simulink model "Example4"  (R2020a)
settings: Solver=ode15s  StartTime=0.0  StopTime=0.2  FixedStep=0.01  RelTol=1e-3
undefined symbols (not defined in the file): b, J, K, L, R
settings Model: DataDictionary=motor_data.sldd  Creator=aishw  LastModifiedBy=aishw

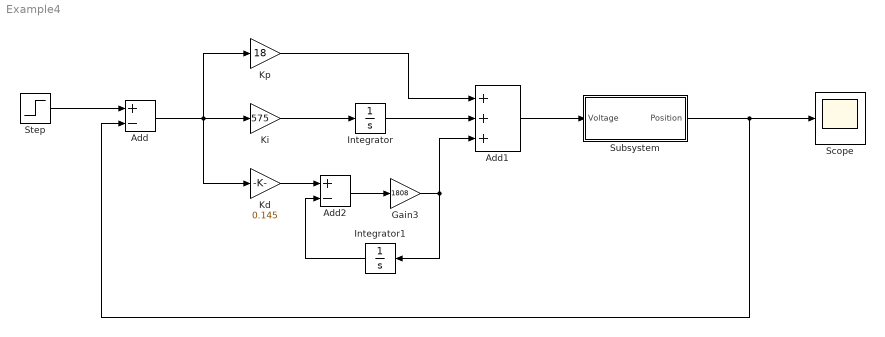
== system Example4 ==
  Add : Sum  Inputs=+-
  Add1 : Sum  Inputs=+++
  Add2 : Sum  Inputs=+-
  Gain3 : Gain  Gain=1808
  Integrator : Integrator
  Integrator1 : Integrator
  Kd : Gain  Gain=0.145
  Ki : Gain  Gain=575
  Kp : Gain  Gain=18
  Scope : Scope
  Step : Step  Time=0  SampleTime=0
  Subsystem : Subsystem  TreatAsAtomicUnit=on
  wires:
  Add1/1 -> Subsystem/1(Voltage)
  Step/1 -> Add/1
  Subsystem/1(Position) -> Add/2, Scope/1
  Add/1 -> Kd/1, Ki/1, Kp/1
  Ki/1 -> Integrator/1
  Kp/1 -> Add1/1
  Integrator/1 -> Add1/2
  Integrator1/1 -> Add2/2
  Kd/1 -> Add2/1
  Gain3/1 -> Add1/3, Integrator1/1
  Add2/1 -> Gain3/1

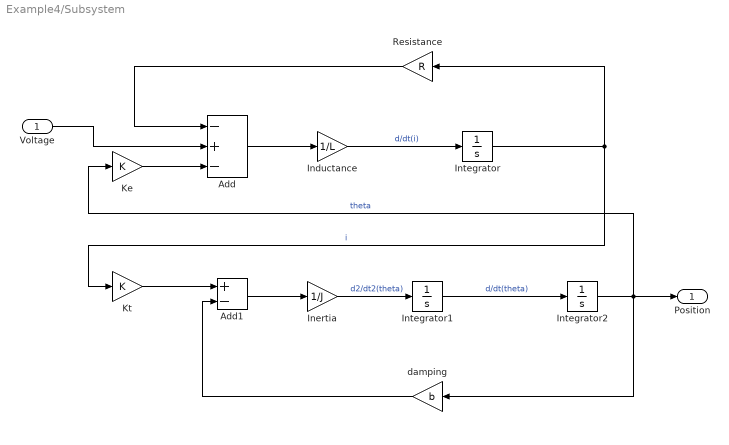
== system Example4/Subsystem ==
  Voltage : Inport
  Add : Sum  Inputs=-+-
  Add1 : Sum  Inputs=+-
  Inductance : Gain  Gain=1/L
  Inertia : Gain  Gain=1/J
  Integrator : Integrator
  Integrator1 : Integrator
  Integrator2 : Integrator
  Ke : Gain  Gain=K
  Kt : Gain  Gain=K
  Resistance : Gain  Gain=R
  damping : Gain  Gain=b
  Position : Outport
  wires:
  Inductance/1 -> Integrator/1  "d/dt(i)"
  Integrator/1 -> Kt/1, Resistance/1  "i"
  Inertia/1 -> Integrator1/1  "d2/dt2(theta)"
  Integrator1/1 -> Integrator2/1  "d/dt(theta)"
  Integrator2/1 -> damping/1, Position/1, Ke/1  "theta"
  Add1/1 -> Inertia/1
  Kt/1 -> Add1/1
  Add/1 -> Inductance/1
  damping/1 -> Add1/2
  Ke/1 -> Add/3
  Resistance/1 -> Add/1
  Voltage/1 -> Add/2
